simulink model "StateComponent"  (R2016a)
settings: Solver=ode45  StartTime=0.0  StopTime=10.0  RelTol=1e-3
settings Model: Creator=sz609516  LastModifiedBy=fhu
settings DataIOCC: LimitDataPoints=on  SaveFormat=Array
settings DebuggingCC: UnderspecifiedInitializationDetection=Classic  MergeDetectMultiDrivingBlocksExec=none  SolverPrmCheckMsg=warning  StateNameClashWarn=warning
settings HardwareCC: ProdBitPerPointer=32  ProdLargestAtomicFloat=None  ProdIntDivRoundTo=Undefined  ProdEndianess=Unspecified  ProdWordSize=32  ProdHWDeviceType=32-bit Generic
settings ModelReferenceCC: PropagateSignalLabelsOutOfModel=off
settings ConfigComp: CovModelRefEnable=Off

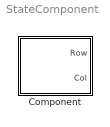
== system StateComponent ==
  Component : Subsystem

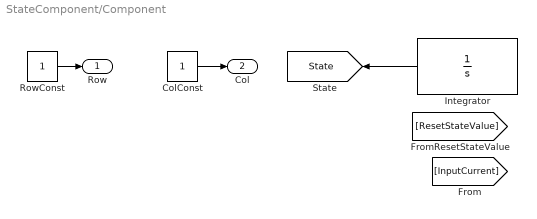
== system StateComponent/Component ==
  ColConst : Constant
  Integrator : Integrator  ExternalReset=either  InitialConditionSource=external
  RowConst : Constant
  Row : Outport
  Col : Outport  Port=2
  tag scope: State=global
  wires:
  RowConst/1 -> Row/1
  ColConst/1 -> Col/1
  Integrator/1 -> [State]
